simulink model "PMSM_Model_2020b"  (R2020b)
settings: Solver=ode23s  StartTime=0.0  StopTime=10  FixedStep=1e-4  MaxStep=1e-4  RelTol=1e-4
model workspace (MAT data in the model file):
  B = 9.557e-05
  J = 2.6e-05
  Ls = 0.0062
  P = 4
  Rs = 1.45
  Tc = 0.03
  Vm = 99.7418632117
  f = 99.6381578947
  lamdaM = 0.062
settings Model: Creator=ahmed  LastModifiedBy=ahmed
settings DebuggingCC: UnconnectedInputMsg=none  UnconnectedOutputMsg=none  UnconnectedLineMsg=none
settings ModelReferenceCC: EnableRefExpFcnMdlSchedulingChecks=off
settings RTWCC: GPUComputeCapability=5.0

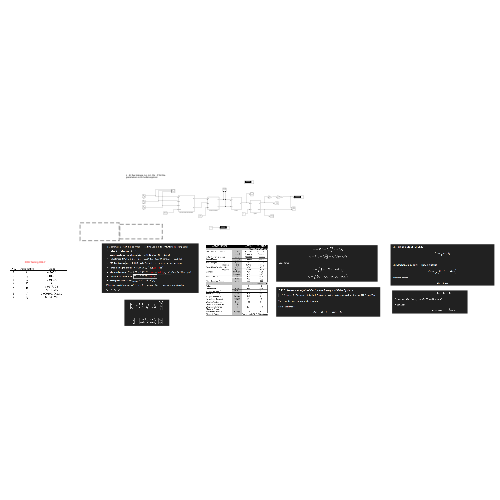
[thumbnail: Simulink's stored preview of the top-level diagram]
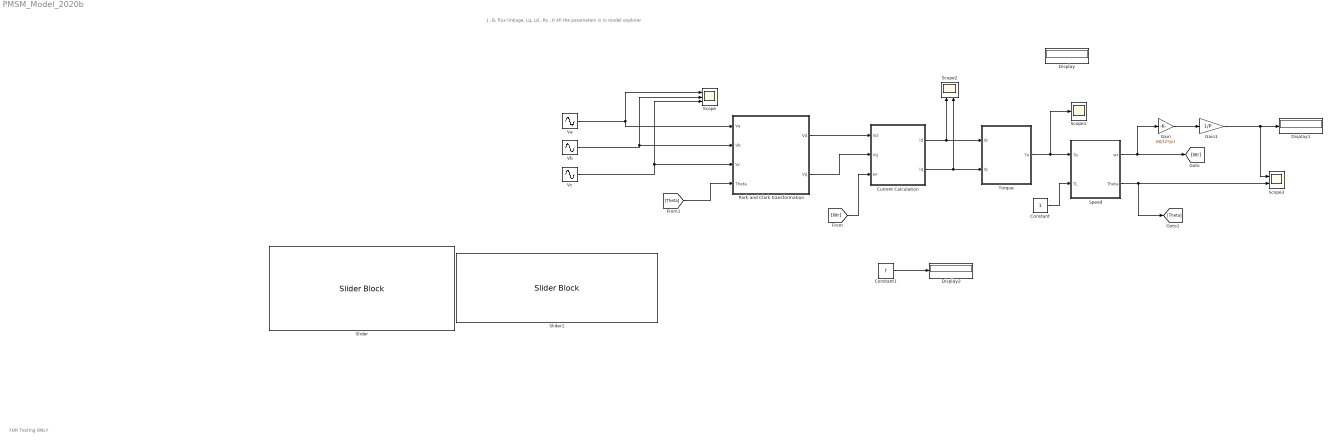
== system PMSM_Model_2020b ==
  note: FOR Testing ONLY
  note: J , B, flux linkage, Lq, Ld , Rs , P All the parameters is in model explorer
  Constant : Constant
  Constant1 : Constant  Value=f
  Current Calculation : Subsystem
  Display : Display
  Display1 : Display
  Display2 : Display
  Gain : Gain  Gain=60/(2*pi)
  Gain1 : Gain  Gain=1/P
  Park and Clark transformation : Subsystem
  Scope : Scope  NumInputPorts=3
  Scope1 : Scope
  Scope2 : Scope  NumInputPorts=2
  Scope3 : Scope  NumInputPorts=2
  Slider : SliderBlock  ScaleMax=325
  Slider1 : SliderBlock  ScaleMax=325
  Speed : Subsystem
  "Torque " : Subsystem
  Va : Sin  Amplitude=Vm  Frequency=2*f*pi  SampleTime=0
  Vb : Sin  Amplitude=Vm  Frequency=2*f*pi  Phase=-(120*(pi/180))  SampleTime=0
  Vc : Sin  Amplitude=Vm  Frequency=2*f*pi  Phase=-(240*(pi/180))  SampleTime=0
  wires:
  Va/1 -> Scope/1, Park and Clark transformation/1(Va)
  Vb/1 -> Scope/2, Park and Clark transformation/2(Vb)
  Vc/1 -> Scope/3, Park and Clark transformation/3(Vc)
  Park and Clark transformation/1(Vd) -> Current Calculation/1(Vd)
  Park and Clark transformation/2(Vq) -> Current Calculation/2(Vq)
  "Torque "/1(Te) -> Scope1/1, Speed/1(Te)
  Speed/1(wr) -> [Wr], Gain/1
  [Wr] -> Current Calculation/3(wr)
  Current Calculation/2(Iq) -> "Torque "/2(Iq), Scope2/2
  Current Calculation/1(Id) -> "Torque "/1(Id), Scope2/1
  Speed/2(Theta) -> [Theta], Scope3/2
  Gain/1 -> Gain1/1
  Gain1/1 -> Scope3/1, Display1/1
  [Theta] -> Park and Clark transformation/4(Theta)
  Constant/1 -> Speed/2(TL)
  Constant1/1 -> Display2/1

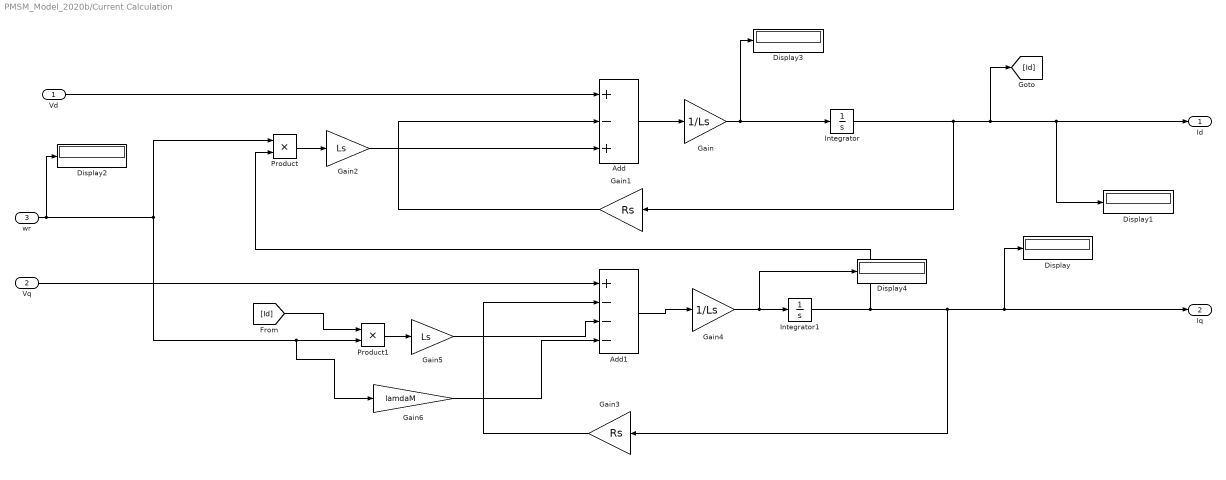
== system PMSM_Model_2020b/Current Calculation ==
  Vd : Inport
  Vq : Inport  Port=2
  wr : Inport  Port=3
  Add : Sum  Inputs=+-+
  Add1 : Sum  Inputs=+---
  Display{,1..4} (5 alike) : Display
  Gain : Gain  Gain=1/Ls
  Gain1 : Gain  Gain=Rs
  Gain2 : Gain  Gain=Ls
  Gain3 : Gain  Gain=Rs
  Gain4 : Gain  Gain=1/Ls
  Gain5 : Gain  Gain=Ls
  Gain6 : Gain  Gain=lamdaM
  Integrator : Integrator
  Integrator1 : Integrator
  Product : Product
  Product1 : Product
  Id : Outport
  Iq : Outport  Port=2
  wires:
  Vd/1 -> Add/1
  Add/1 -> Gain/1
  Gain/1 -> Integrator/1, Display3/1
  Integrator/1 -> Gain1/1, [Id], Display1/1, Id/1
  Gain1/1 -> Add/2
  wr/1 -> Product/1, Gain6/1, Product1/2, Display2/1
  Product/1 -> Gain2/1
  Gain2/1 -> Add/3
  Vq/1 -> Add1/1
  Add1/1 -> Gain4/1
  Gain4/1 -> Display4/1, Integrator1/1
  Integrator1/1 -> Product/2, Display/1, Iq/1, Gain3/1
  Gain3/1 -> Add1/2
  [Id] -> Product1/1
  Product1/1 -> Gain5/1
  Gain5/1 -> Add1/3
  Gain6/1 -> Add1/4

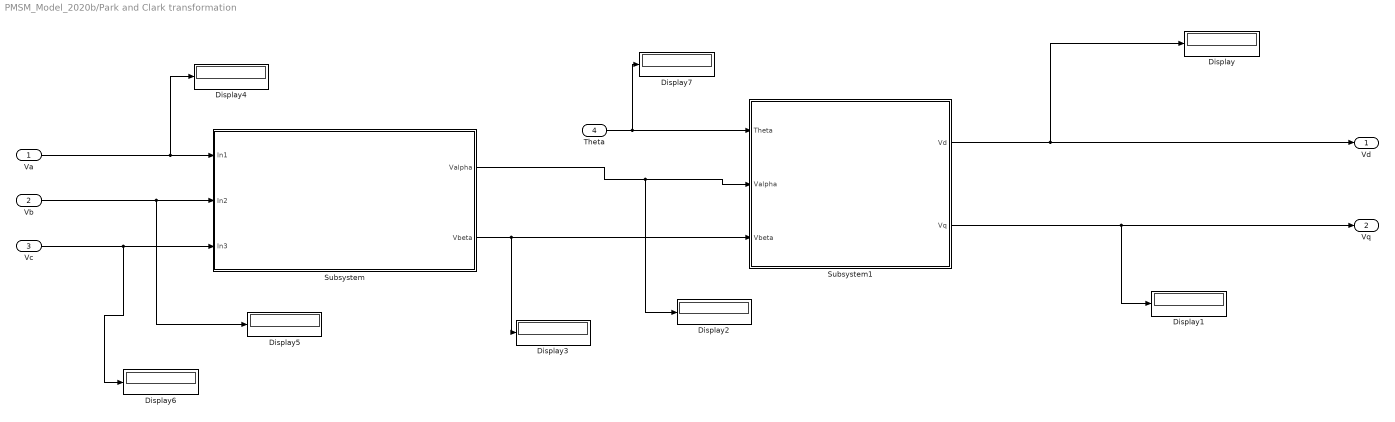
== system PMSM_Model_2020b/Park and Clark transformation ==
  Va : Inport
  Vb : Inport  Port=2
  Vc : Inport  Port=3
  Theta : Inport  Port=4
  Display{,1..7} (8 alike) : Display
  Subsystem : Subsystem
  Subsystem1 : Subsystem
  Vd : Outport
  Vq : Outport  Port=2
  wires:
  Va/1 -> Display4/1, Subsystem/1(In1)
  Vb/1 -> Display5/1, Subsystem/2(In2)
  Vc/1 -> Display6/1, Subsystem/3(In3)
  Subsystem/1(Valpha) -> Display2/1, Subsystem1/2(Valpha)
  Subsystem/2(Vbeta) -> Display3/1, Subsystem1/3(Vbeta)
  Subsystem1/1(Vd) -> Display/1, Vd/1
  Subsystem1/2(Vq) -> Vq/1, Display1/1
  Theta/1 -> Display7/1, Subsystem1/1(Theta)

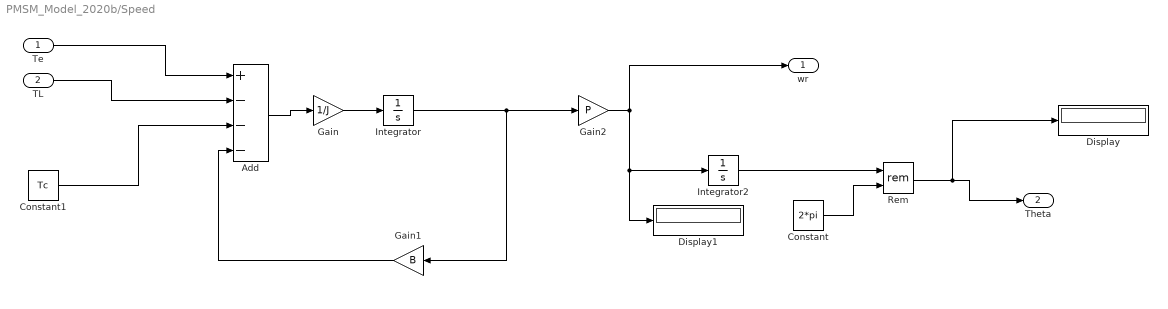
== system PMSM_Model_2020b/Speed ==
  Te : Inport
  TL : Inport  Port=2
  Add : Sum  Inputs=+---
  Constant : Constant  Value=2*pi
  Constant1 : Constant  Value=Tc
  Display : Display
  Display1 : Display
  Gain : Gain  Gain=1/J
  Gain1 : Gain  Gain=B
  Gain2 : Gain  Gain=P
  Integrator : Integrator
  Integrator2 : Integrator
  Rem : Math  Operator=rem  SaturateOnIntegerOverflow=on
  wr : Outport
  Theta : Outport  Port=2
  wires:
  Te/1 -> Add/1
  Gain/1 -> Integrator/1
  TL/1 -> Add/2
  Add/1 -> Gain/1
  Gain1/1 -> Add/4
  Integrator/1 -> Gain1/1, Gain2/1
  Gain2/1 -> Display1/1, Integrator2/1, wr/1
  Integrator2/1 -> Rem/1
  Constant/1 -> Rem/2
  Rem/1 -> Display/1, Theta/1
  Constant1/1 -> Add/3

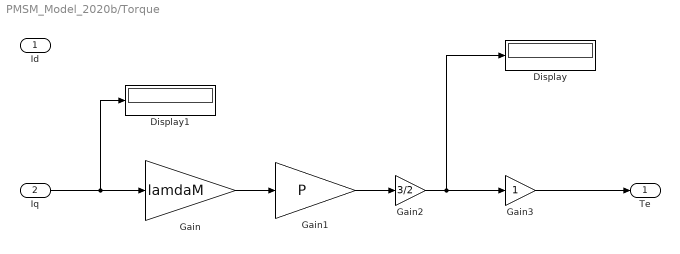
== system PMSM_Model_2020b/Torque  ==
  Id : Inport
  Iq : Inport  Port=2
  Display : Display
  Display1 : Display
  Gain : Gain  Gain=lamdaM
  Gain1 : Gain  Gain=P
  Gain2 : Gain  Gain=3/2
  Gain3 : Gain
  Te : Outport
  wires:
  Iq/1 -> Display1/1, Gain/1
  Gain/1 -> Gain1/1
  Gain2/1 -> Display/1, Gain3/1
  Gain1/1 -> Gain2/1
  Gain3/1 -> Te/1

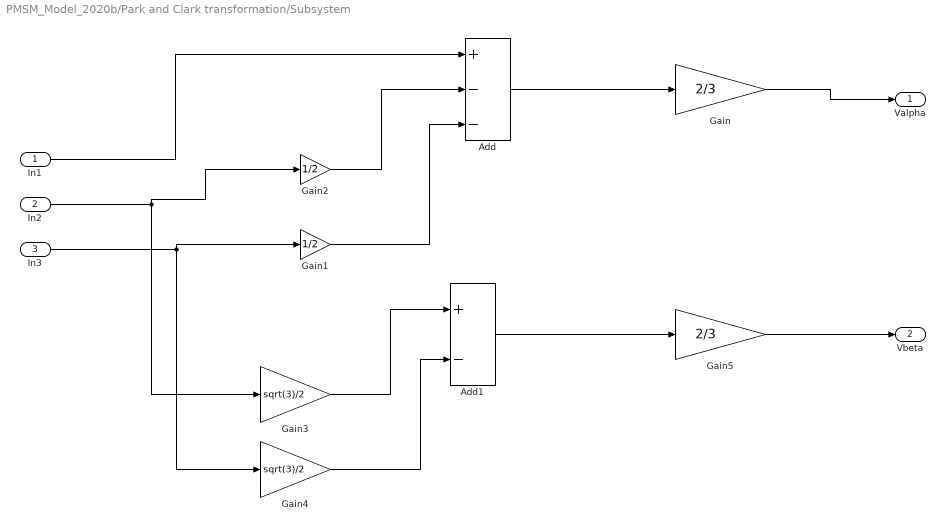
== system PMSM_Model_2020b/Park and Clark transformation/Subsystem ==
  In1 : Inport
  In2 : Inport  Port=2
  In3 : Inport  Port=3
  Add : Sum  Inputs=+--
  Add1 : Sum  Inputs=+-
  Gain : Gain  Gain=2/3
  Gain1 : Gain  Gain=1/2
  Gain2 : Gain  Gain=1/2
  Gain3 : Gain  Gain=sqrt(3)/2
  Gain4 : Gain  Gain=sqrt(3)/2
  Gain5 : Gain  Gain=2/3
  Valpha : Outport
  Vbeta : Outport  Port=2
  wires:
  Gain3/1 -> Add1/1
  Gain1/1 -> Add/3
  Gain2/1 -> Add/2
  In2/1 -> Gain2/1, Gain3/1
  Gain5/1 -> Vbeta/1
  Gain4/1 -> Add1/2
  In3/1 -> Gain1/1, Gain4/1
  Add/1 -> Gain/1
  Add1/1 -> Gain5/1
  Gain/1 -> Valpha/1
  In1/1 -> Add/1

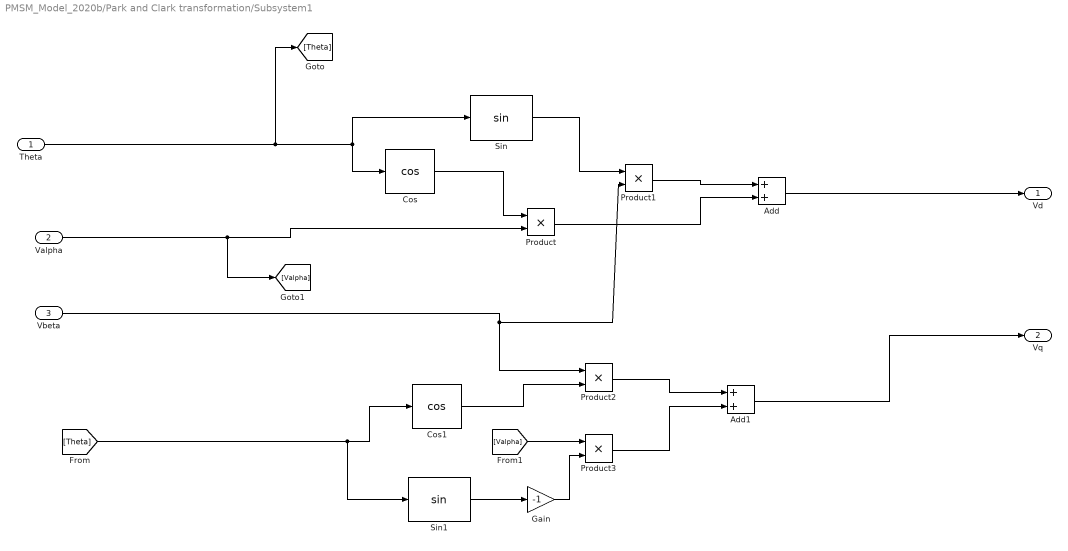
== system PMSM_Model_2020b/Park and Clark transformation/Subsystem1 ==
  Theta : Inport
  Valpha : Inport  Port=2
  Vbeta : Inport  Port=3
  Add : Sum
  Add1 : Sum
  Cos : Trigonometry  Operator=cos
  Cos1 : Trigonometry  Operator=cos
  Gain : Gain  Gain=-1
  Product{,1..3} (4 alike) : Product
  Sin : Trigonometry
  Sin1 : Trigonometry
  Vd : Outport
  Vq : Outport  Port=2
  wires:
  Sin1/1 -> Gain/1
  Gain/1 -> Product3/2
  Product/1 -> Add/2
  Sin/1 -> Product1/1
  Theta/1 -> [Theta], Cos/1, Sin/1
  Product1/1 -> Add/1
  [Theta] -> Sin1/1, Cos1/1
  Cos1/1 -> Product2/2
  Cos/1 -> Product/1
  Product3/1 -> Add1/2
  Product2/1 -> Add1/1
  Vbeta/1 -> Product2/1, Product1/2
  [Valpha] -> Product3/1
  Add/1 -> Vd/1
  Valpha/1 -> [Valpha], Product/2
  Add1/1 -> Vq/1
